simulink model "ANC_simulink_4"  (R2023b)
settings: Solver=VariableStepAuto  StartTime=0.0  StopTime=1  RelTol=1e-3
values from neighbouring files (symbols this model uses):
  A = 10    [parameter.mat]
  c = 343    [parameter.mat]
  f = 10    [parameter.mat]
  Lp = 1    [parameter.mat]
  Ls = 0.1    [parameter.mat]
  Ts = 0.001    [parameter.mat]
settings Model: Creator=nurbi  LastModifiedBy=nurbi

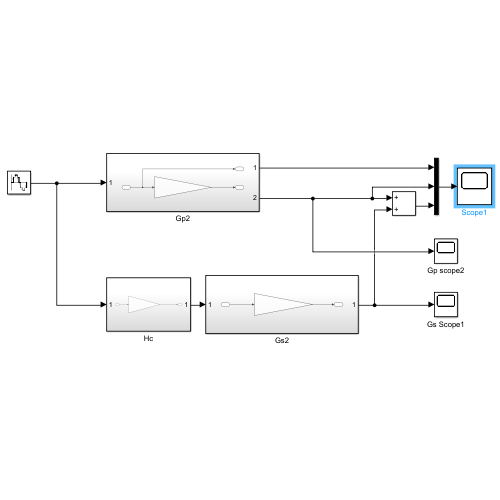
[thumbnail: Simulink's stored preview of the top-level diagram]
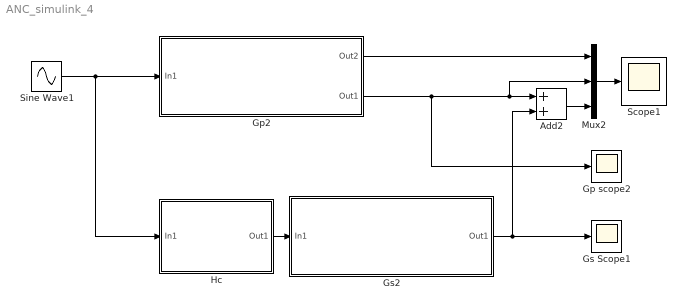
== system ANC_simulink_4 ==
  Add2 : Sum
  Gp scope2 : Scope
  Gp2 : Subsystem
  Gs Scope1 : Scope
  Gs2 : Subsystem
  Hc : Subsystem
  Mux2 : Mux  Inputs=3
  Scope1 : Scope
  Sine Wave1 : Sin  Amplitude=A  Frequency=2*pi*f  SampleTime=Ts
  wires:
  Mux2/1 -> Scope1/1
  Gs2/1(Out1) -> Add2/2, Gs Scope1/1
  Sine Wave1/1 -> Hc/1(In1), Gp2/1(In1)
  Gp2/2(Out1) -> Add2/1, Mux2/2, Gp scope2/1
  Hc/1(Out1) -> Gs2/1(In1)
  Gp2/1(Out2) -> Mux2/1
  Add2/1 -> Mux2/3

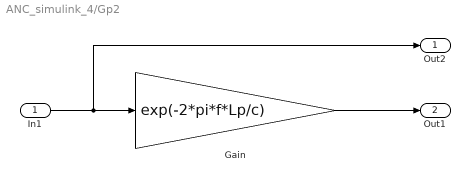
== system ANC_simulink_4/Gp2 ==
  In1 : Inport
  Gain : Gain  Gain=exp(-2*pi*f*Lp/c)
  Out2 : Outport
  Out1 : Outport  Port=2
  wires:
  In1/1 -> Gain/1, Out2/1
  Gain/1 -> Out1/1

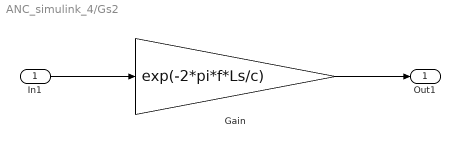
== system ANC_simulink_4/Gs2 ==
  In1 : Inport
  Gain : Gain  Gain=exp(-2*pi*f*Ls/c)
  Out1 : Outport
  wires:
  In1/1 -> Gain/1
  Gain/1 -> Out1/1

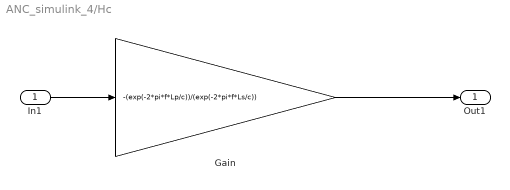
== system ANC_simulink_4/Hc ==
  In1 : Inport
  Gain : Gain  Gain=-(exp(-2*pi*f*Lp/c))/(exp(-2*pi*f*Ls/c))
  Out1 : Outport
  wires:
  Gain/1 -> Out1/1
  In1/1 -> Gain/1
